simulink model "li_slotine"  (R2020b)
settings: Solver=VariableStepAuto  StartTime=0.0  StopTime=80  RelTol=1e-3
InitFcn:
  | UR5_LI_SLOTINE
values from neighbouring files (symbols this model uses):
  init_cond_regress = zeros(60, 1)    [UR5_LI_SLOTINE.m]    (also in parametersUR5_ADAPTIVE_BACKSTEPPING.m)
  init_config = [0,-55.5,-131,-2.5,20,105]'*pi/180    [UR5_LI_SLOTINE.m]    (also in parametersUR5_ADAPTIVE_BACKSTEPPING.m = [0,-37,-110,-2.5,-1,55]'*pi/180; parametersUR5_BACKSTEPPING.m = [0,-37,-110,-2.5,-1,55]'*pi/180)
  m1 = ur5.links(1,1).m    [UR5_LI_SLOTINE.m]    (also in parametersUR5_ADAPTIVE_BACKSTEPPING.m; parametersUR5_BACKSTEPPING.m)
  m2 = ur5.links(1,2).m    [UR5_LI_SLOTINE.m]    (also in parametersUR5_ADAPTIVE_BACKSTEPPING.m; parametersUR5_BACKSTEPPING.m)
  m3 = ur5.links(1,3).m    [UR5_LI_SLOTINE.m]    (also in parametersUR5_ADAPTIVE_BACKSTEPPING.m; parametersUR5_BACKSTEPPING.m)
  m4 = ur5.links(1,4).m    [UR5_LI_SLOTINE.m]    (also in parametersUR5_ADAPTIVE_BACKSTEPPING.m; parametersUR5_BACKSTEPPING.m)
  m5 = ur5.links(1,5).m    [UR5_LI_SLOTINE.m]    (also in parametersUR5_ADAPTIVE_BACKSTEPPING.m; parametersUR5_BACKSTEPPING.m)
  m6 = ur5.links(1,6).m    [UR5_LI_SLOTINE.m]    (also in parametersUR5_ADAPTIVE_BACKSTEPPING.m; parametersUR5_BACKSTEPPING.m)
  Ts = 1/100    (= 0.01)    [UR5_LI_SLOTINE.m]    (also in parametersUR5_ADAPTIVE_BACKSTEPPING.m; parametersUR5_BACKSTEPPING.m)
libraries: simulink x3, robotcorelib x1, cstblocks x1
settings Model: Creator=stefa  LastModifiedBy=stefa

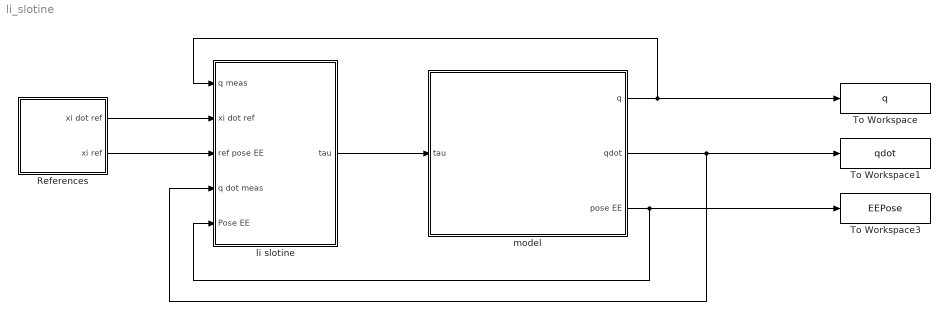
== system li_slotine ==
  References : Subsystem
  To Workspace : ToWorkspace  VariableName=q  SaveFormat=Timeseries  SampleTime=Ts
  To Workspace1 : ToWorkspace  VariableName=qdot  SaveFormat=Timeseries  SampleTime=Ts
  To Workspace3 : ToWorkspace  VariableName=EEPose  SaveFormat=Timeseries  SampleTime=Ts
  li slotine : Subsystem  StopFcn=show_results
  model : Subsystem
  wires:
  li slotine/1(tau) -> model/1(tau)
  model/1(q) -> li slotine/1(q meas), To Workspace/1
  model/2(qdot) -> li slotine/4(q dot meas), To Workspace1/1
  model/3(pose EE) -> li slotine/5(Pose EE), To Workspace3/1
  References/2(xi ref) -> li slotine/3(ref pose EE)
  References/1(xi dot ref) -> li slotine/2(xi dot ref)

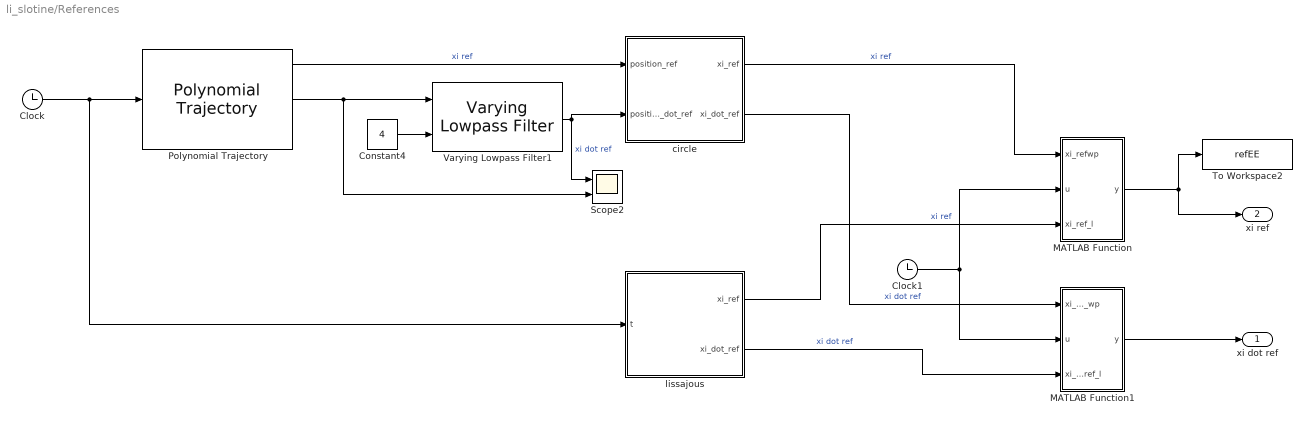
== system li_slotine/References ==
  Clock : Clock
  Clock1 : Clock
  Constant4 : Constant  Value=4
  MATLAB Function : MATLAB Function  TreatAsAtomicUnit=on
  MATLAB Function1 : MATLAB Function  TreatAsAtomicUnit=on
  Polynomial Trajectory : robotcorelib/Polynomial Trajectory  WaypointSource=Internal  Waypoints=waypoints  TimePoints=timepoints  TimeInterval=[ 1, 4 ]  Method=Cubic Polynomial  ParameterSource=Internal  VelocityBoundaryCondition=velocitybc  AccelerationBoundaryCondition=zeros( 2, 5 )  SimulateUsing=Interpreted execution
  Scope2 : Scope  NumInputPorts=2
  To Workspace2 : ToWorkspace  VariableName=refEE  SaveFormat=Timeseries  SampleTime=Ts
  Varying Lowpass Filter1 : cstblocks/Linear Parameter Varying/Varying Lowpass Filter  N=1
  circle : MATLAB Function  TreatAsAtomicUnit=on
  lissajous : MATLAB Function  TreatAsAtomicUnit=on
  xi dot ref : Outport
  xi ref : Outport  Port=2
  wires:
  lissajous/2(xi_dot_ref) -> MATLAB Function1/3(xi_dot_ref_l)  "xi dot ref"
  Polynomial Trajectory/2 -> Scope2/2, Varying Lowpass Filter1/1
  Constant4/1 -> Varying Lowpass Filter1/2
  circle/2(xi_dot_ref) -> MATLAB Function1/1(xi_dot_ref_wp)  "xi dot ref"
  Varying Lowpass Filter1/1 -> Scope2/1, circle/2(position_dot_ref)  "xi dot ref"
  circle/1(xi_ref) -> MATLAB Function/1(xi_refwp)  "xi ref"
  Clock/1 -> lissajous/1(t), Polynomial Trajectory/1
  Polynomial Trajectory/1 -> circle/1(position_ref)  "xi ref"
  lissajous/1(xi_ref) -> MATLAB Function/3(xi_ref_l)  "xi ref"
  MATLAB Function/1(y) -> xi ref/1, To Workspace2/1
  MATLAB Function1/1(y) -> xi dot ref/1
  Clock1/1 -> MATLAB Function1/2(u), MATLAB Function/2(u)

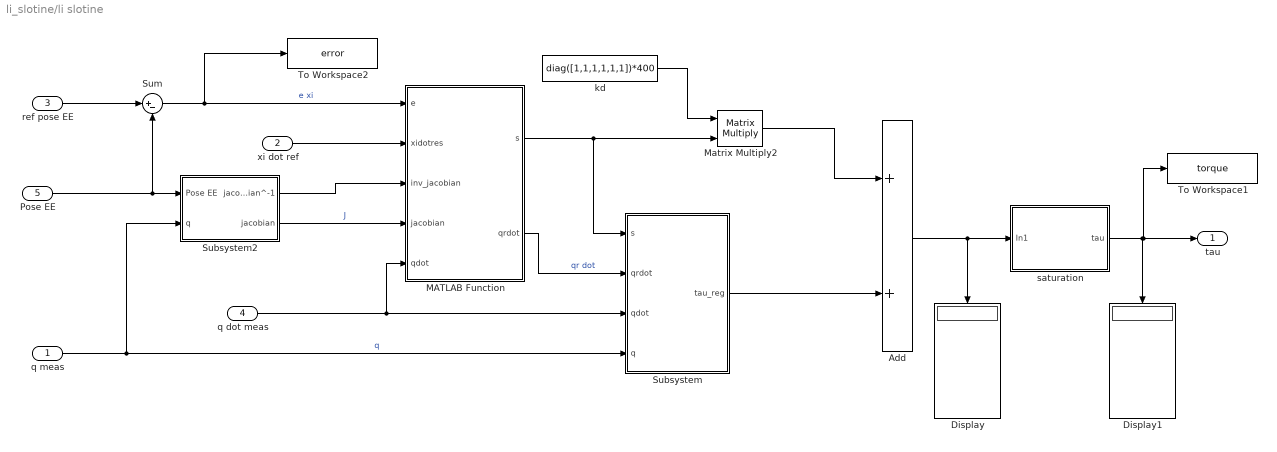
== system li_slotine/li slotine ==
  q meas : Inport
  xi dot ref : Inport  Port=2
  ref pose EE : Inport  Port=3
  q dot meas : Inport  Port=4
  Pose EE : Inport  Port=5
  Add : Sum
  Display : Display
  Display1 : Display
  MATLAB Function : MATLAB Function  TreatAsAtomicUnit=on
  Matrix Multiply2 : Product  Multiplication=Matrix(*)
  Subsystem : Subsystem
  Subsystem2 : Subsystem
  Sum : Sum  Inputs=|+-
  To Workspace1 : ToWorkspace  VariableName=torque  SaveFormat=Timeseries  SampleTime=Ts
  To Workspace2 : ToWorkspace  VariableName=error  SaveFormat=Timeseries  SampleTime=Ts
  kd : Constant  Value=diag([1,1,1,1,1,1])*400
  saturation : Subsystem
  tau : Outport
  wires:
  Add/1 -> saturation/1(In1), Display/1
  q meas/1 -> Subsystem/4(q), Subsystem2/2(q)  "q"
  MATLAB Function/2(qrdot) -> Subsystem/2(qrdot)  "qr dot"
  q dot meas/1 -> Subsystem/3(qdot), MATLAB Function/5(qdot)
  ref pose EE/1 -> Sum/1
  Pose EE/1 -> Sum/2, Subsystem2/1(Pose EE)
  Sum/1 -> To Workspace2/1, MATLAB Function/1(e)  "e xi"
  Subsystem2/1(jacobian^-1) -> MATLAB Function/3(inv_jacobian)
  Subsystem2/2(jacobian) -> MATLAB Function/4(jacobian)  "J"
  MATLAB Function/1(s) -> Subsystem/1(s), Matrix Multiply2/2
  Matrix Multiply2/1 -> Add/1
  kd/1 -> Matrix Multiply2/1
  xi dot ref/1 -> MATLAB Function/2(xidotres)
  Subsystem/1(tau_reg) -> Add/2
  saturation/1(tau) -> tau/1, To Workspace1/1, Display1/1

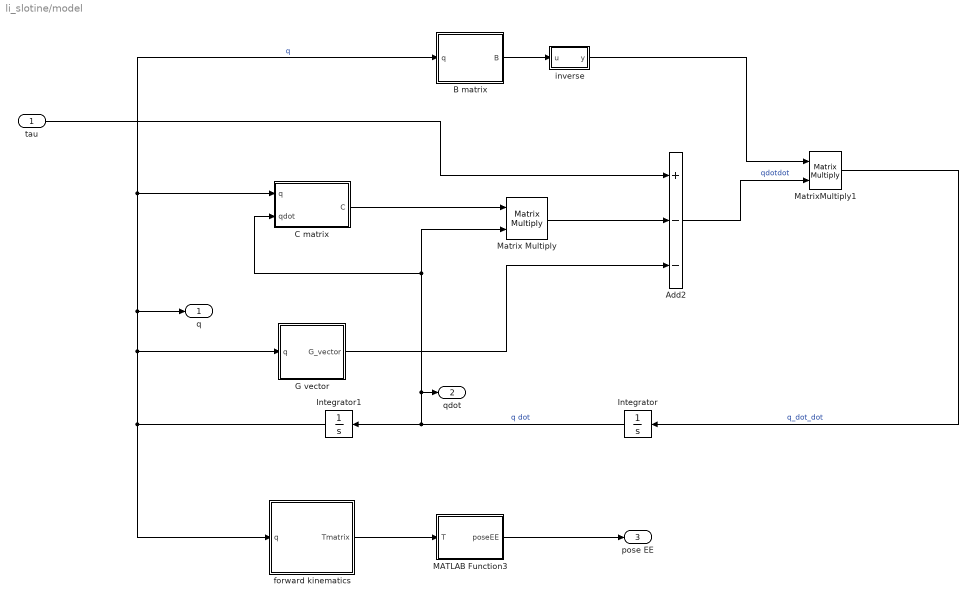
== system li_slotine/model ==
  tau : Inport
  Add2 : Sum  Inputs=+--
  B matrix : MATLAB Function  TreatAsAtomicUnit=on
  C matrix : MATLAB Function  TreatAsAtomicUnit=on
  G vector : MATLAB Function  TreatAsAtomicUnit=on
  Integrator : Integrator  InitialCondition=[0,0,0,0,0,0]'
  Integrator1 : Integrator  InitialCondition=init_config
  MATLAB Function3 : MATLAB Function  TreatAsAtomicUnit=on
  Matrix Multiply : Product  Multiplication=Matrix(*)
  MatrixMultiply1 : Product  Multiplication=Matrix(*)
  forward kinematics : MATLAB Function  TreatAsAtomicUnit=on
  inverse : MATLAB Function  TreatAsAtomicUnit=on
  q : Outport
  qdot : Outport  Port=2
  pose EE : Outport  Port=3
  wires:
  MatrixMultiply1/1 -> Integrator/1  "q_dot_dot"
  B matrix/1(B) -> inverse/1(u)
  inverse/1(y) -> MatrixMultiply1/1
  tau/1 -> Add2/1
  Matrix Multiply/1 -> Add2/2
  C matrix/1(C) -> Matrix Multiply/1
  Integrator/1 -> C matrix/2(qdot), Matrix Multiply/2, qdot/1, Integrator1/1  "q dot"
  Integrator1/1 -> G vector/1(q), q/1, B matrix/1(q), C matrix/1(q), forward kinematics/1(q)  "q"
  G vector/1(G_vector) -> Add2/3
  Add2/1 -> MatrixMultiply1/2  "qdotdot"
  forward kinematics/1(Tmatrix) -> MATLAB Function3/1(T)
  MATLAB Function3/1(poseEE) -> pose EE/1

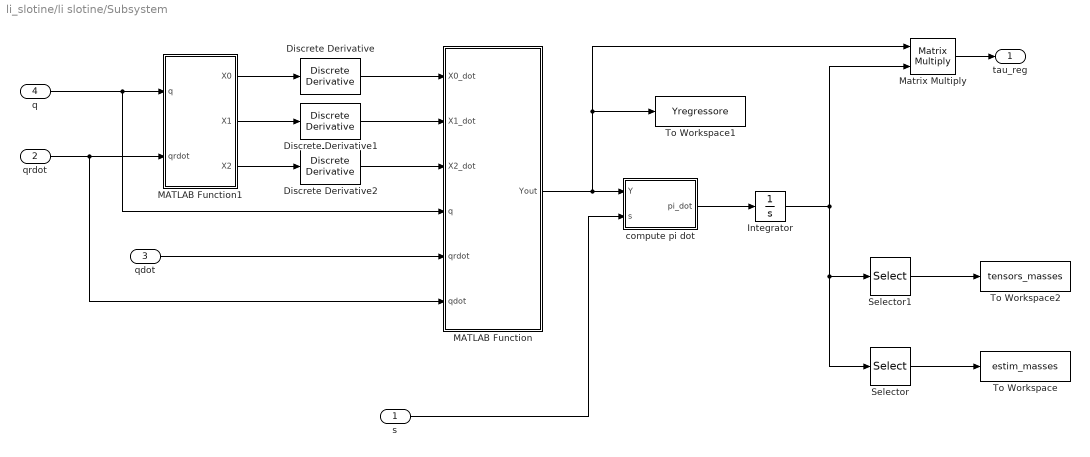
== system li_slotine/li slotine/Subsystem ==
  s : Inport
  qrdot : Inport  Port=2
  qdot : Inport  Port=3
  q : Inport  Port=4
  Discrete Derivative : simulink/Discrete/Discrete Derivative  gainval=1.0  ICPrevScaledInput=0.0  OutMin=[]  OutMax=[]  OutDataType=fixdt(1, 16)  OutScaling=2^-10  DoSatur=off
  Discrete Derivative1 : simulink/Discrete/Discrete Derivative  gainval=1.0  ICPrevScaledInput=0.0  OutMin=[]  OutMax=[]  OutDataType=fixdt(1, 16)  OutScaling=2^-10  DoSatur=off
  Discrete Derivative2 : simulink/Discrete/Discrete Derivative  gainval=1.0  ICPrevScaledInput=0.0  OutMin=[]  OutMax=[]  OutDataType=fixdt(1, 16)  OutScaling=2^-10  DoSatur=off
  Integrator : Integrator  InitialCondition=init_cond_regress
  MATLAB Function : MATLAB Function  TreatAsAtomicUnit=on
  MATLAB Function1 : MATLAB Function  TreatAsAtomicUnit=on
  Matrix Multiply : Product  Multiplication=Matrix(*)
  Selector : Selector  InputPortWidth=60  IndexOptions=Index vector (dialog)  Indices=[1:6]  OutputSizes=1
  Selector1 : Selector  InputPortWidth=60  IndexOptions=Index vector (dialog)  Indices=[25:60]  OutputSizes=1
  To Workspace : ToWorkspace  VariableName=estim_masses  SaveFormat=Timeseries  SampleTime=Ts
  To Workspace1 : ToWorkspace  VariableName=Yregressore  SaveFormat=Timeseries  SampleTime=Ts
  To Workspace2 : ToWorkspace  VariableName=tensors_masses  SaveFormat=Timeseries  SampleTime=Ts
  compute pi dot : MATLAB Function  TreatAsAtomicUnit=on
  tau_reg : Outport
  wires:
  q/1 -> MATLAB Function/4(q), MATLAB Function1/1(q)
  qrdot/1 -> MATLAB Function/6(qdot), MATLAB Function1/2(qrdot)
  MATLAB Function1/1(X0) -> Discrete Derivative/1
  MATLAB Function1/2(X1) -> Discrete Derivative1/1
  MATLAB Function1/3(X2) -> Discrete Derivative2/1
  Discrete Derivative/1 -> MATLAB Function/1(X0_dot)
  Discrete Derivative1/1 -> MATLAB Function/2(X1_dot)
  Discrete Derivative2/1 -> MATLAB Function/3(X2_dot)
  qdot/1 -> MATLAB Function/5(qrdot)
  MATLAB Function/1(Yout) -> Matrix Multiply/1, To Workspace1/1, compute pi dot/1(Y)
  compute pi dot/1(pi_dot) -> Integrator/1
  s/1 -> compute pi dot/2(s)
  Integrator/1 -> Selector/1, Selector1/1, Matrix Multiply/2
  Matrix Multiply/1 -> tau_reg/1
  Selector/1 -> To Workspace/1
  Selector1/1 -> To Workspace2/1

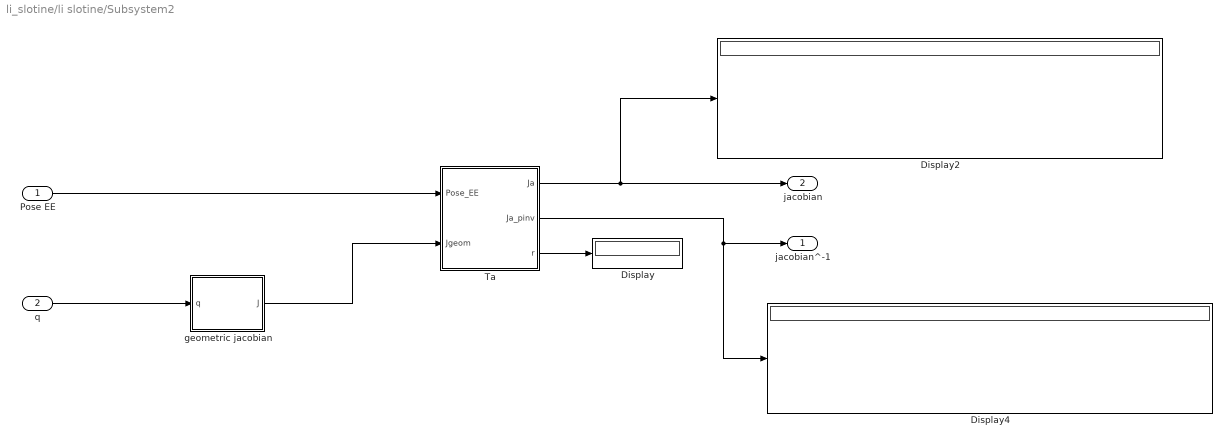
== system li_slotine/li slotine/Subsystem2 ==
  Pose EE : Inport
  q : Inport  Port=2
  Display : Display
  Display2 : Display
  Display4 : Display
  Ta : MATLAB Function  TreatAsAtomicUnit=on
  geometric jacobian : MATLAB Function  TreatAsAtomicUnit=on
  jacobian^-1 : Outport
  jacobian : Outport  Port=2
  wires:
  Pose EE/1 -> Ta/1(Pose_EE)
  q/1 -> geometric jacobian/1(q)
  Ta/2(Ja_pinv) -> jacobian^-1/1, Display4/1
  Ta/1(Ja) -> jacobian/1, Display2/1
  Ta/3(r) -> Display/1
  geometric jacobian/1(J) -> Ta/2(Jgeom)

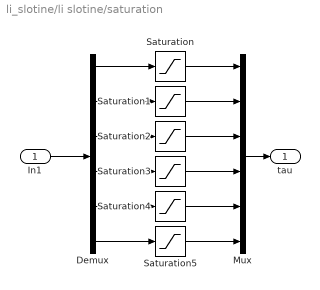
== system li_slotine/li slotine/saturation ==
  In1 : Inport
  Demux : Demux  Outputs=6
  Mux : Mux  Inputs=6
  Saturation : Saturate  UpperLimit=150  LowerLimit=-150
  Saturation1 : Saturate  UpperLimit=150  LowerLimit=-150
  Saturation2 : Saturate  UpperLimit=150  LowerLimit=-150
  Saturation3 : Saturate  UpperLimit=28  LowerLimit=-28
  Saturation4 : Saturate  UpperLimit=28  LowerLimit=-28
  Saturation5 : Saturate  UpperLimit=28  LowerLimit=-28
  tau : Outport
  wires:
  In1/1 -> Demux/1
  Mux/1 -> tau/1
  Demux/1 -> Saturation/1
  Demux/2 -> Saturation1/1
  Demux/3 -> Saturation2/1
  Demux/4 -> Saturation3/1
  Demux/5 -> Saturation4/1
  Demux/6 -> Saturation5/1
  Saturation/1 -> Mux/1
  Saturation1/1 -> Mux/2
  Saturation2/1 -> Mux/3
  Saturation3/1 -> Mux/4
  Saturation4/1 -> Mux/5
  Saturation5/1 -> Mux/6

== matlab function li_slotine/model/forward kinematics ==
  data: q input; Tmatrix output
function Tmatrix = fkine(q)
%#codegen

%    This function was generated by the Symbolic Math Toolbox version 8.6.
%    20-Jan-2022 14:28:01

q1 = q(1);
q2 = q(2);
q3 = q(3);
q4 = q(4);
q5 = q(5);
q6 = q(6);
t2 = cos(q1);
t3 = cos(q2);
t4 = cos(q3);
t5 = cos(q4);
t6 = cos(q5);
t7 = cos(q6);
t8 = sin(q1);
t9 = sin(q2);
t10 = sin(q3);
t11 = sin(q4);
t12 = sin(q5);
t13 = sin(q6);
t14 = q2+q3;
t23 = cos(1.570796327);
t24 = sin(1.570796327);
t25 = sin(3.141592654);
t15 = q4+t14;
t16 = t2.*t3;
t18 = t2.*t9;
t19 = t3.*t8;
t21 = t8.*t9;
t26 = t23.^2;
t27 = t24.^2;
t58 = t2.*t23.*t24;
t59 = t8.*t23.*t24;
t17 = cos(t15);
t20 = sin(t15);
t28 = t16.*t23;
t29 = t18.*t23;
t30 = t19.*t23;
t31 = t21.*t23;
t32 = t2.*t27;
t33 = t8.*t27;
t38 = t3.*t4.*t5.*t27;
t39 = t3.*t10.*t11.*t27;
t40 = t4.*t9.*t11.*t27;
t41 = t5.*t9.*t10.*t27;
t60 = -t58;
t22 = t17+1.0;
t34 = -t28;
t35 = -t31;
t36 = -t33;
t37 = t6.*t20.*t24;
t42 = -t38;
t43 = t18+t30;
t44 = t19+t29;
t61 = t12.*t20.*t23.*t24;
t45 = t16+t35;
t46 = t21+t34;
t47 = (t12.*t22.*t25)./2.0;
t48 = t4.*t43;
t49 = t4.*t44;
t50 = t10.*t43;
t51 = t10.*t44;
t62 = (t6.*t22.*t23.*t25)./2.0;
t85 = t26+t39+t40+t41+t42;
t52 = t4.*t45;
t53 = t4.*t46;
t54 = t10.*t45;
t55 = t10.*t46;
t56 = -t50;
t63 = -t62;
t64 = t37+t47;
t89 = t24.*t85;
t57 = -t55;
t65 = t48+t54;
t66 = t51+t53;
t68 = t52+t56;
t72 = -t5.*(t50-t52);
t80 = -t11.*t23.*(t50-t52);
t82 = -t11.*t24.*(t50-t52);
t103 = t61+t63+t89;
t67 = t49+t57;
t69 = t11.*t65;
t70 = t11.*t66;
t75 = t5.*t23.*t65;
t76 = t5.*t23.*t66;
t77 = t5.*t24.*t65;
t78 = t5.*t24.*t66;
t71 = t5.*t67;
t73 = -t69;
t74 = -t70;
t79 = t11.*t23.*t67;
t81 = t11.*t24.*t67;
t87 = -t6.*(t69+t5.*(t50-t52));
t91 = -t12.*t23.*(t69+t5.*(t50-t52));
t93 = t36+t75+t80;
t97 = t59+t77+t82;
t83 = t71+t74;
t84 = t72+t73;
t86 = -t6.*(t70-t71);
t88 = t6.*(t70-t71);
t90 = -t12.*t23.*(t70-t71);
t92 = t32+t76+t79;
t95 = t12.*t93;
t98 = t60+t78+t81;
t100 = t6.*t23.*t93;
t101 = t24.*t97;
t94 = t12.*t92;
t96 = -t95;
t99 = t6.*t23.*t92;
t102 = t24.*t98;
t107 = t91+t100+t101;
t104 = t88+t94;
t105 = t87+t96;
t106 = t90+t99+t102;
Tmatrix = reshape([-t13.*t107-t7.*(t95+t6.*(t69+t5.*(t50-t52))),-t7.*t104-t13.*t106,t7.*t64-t13.*t103,0.0,-t7.*t107+t13.*(t95+t6.*(t69+t5.*(t50-t52))),-t7.*t106+t13.*t104,-t13.*t64-t7.*t103,0.0,t23.*t97+t12.*t24.*(t69+t5.*(t50-t52))-t6.*t24.*t93,t23.*t98-t6.*t24.*t92+t12.*t24.*(t70-t71),t23.*t85-t12.*t20.*t27+(t6.*t22.*t24.*t25)./2.0,0.0,t16.*(-1.7e+1./4.0e+1)+t31.*(1.7e+1./4.0e+1)+t50.*3.9225e-1-t52.*3.9225e-1+t59.*9.465e-2+t77.*9.465e-2+t8.*t24.*1.0915e-1+t23.*t97.*8.23e-2+t12.*t24.*(t69+t5.*(t50-t52)).*8.23e-2-t6.*t24.*t93.*8.23e-2-t11.*t24.*(t50-t52).*9.465e-2,t19.*(-1.7e+1./4.0e+1)-t29.*(1.7e+1./4.0e+1)-t49.*3.9225e-1+t55.*3.9225e-1-t58.*9.465e-2+t78.*9.465e-2+t81.*9.465e-2-t2.*t24.*1.0915e-1+t23.*t98.*8.23e-2-t6.*t24.*t92.*8.23e-2+t12.*t24.*(t70-t71).*8.23e-2,t23.*1.0915e-1+t26.*9.465e-2-t9.*t24.*(1.7e+1./4.0e+1)-t23.*t38.*8.23e-2+t23.*t39.*8.23e-2+t23.*t40.*8.23e-2+t23.*t41.*8.23e-2+t23.^3.*8.23e-2-t5.*t27.*cos(t14).*9.465e-2+t11.*t27.*sin(t14).*9.465e-2-t3.*t10.*t24.*3.9225e-1-t4.*t9.*t24.*3.9225e-1+t6.*t24.*t25.*4.115e-2-t12.*t20.*t27.*8.23e-2+t6.*t17.*t24.*t25.*4.115e-2+8.9459e-2,1.0],[4,4]);

== matlab function li_slotine/li slotine/Subsystem2/Ta ==
  data: Pose_EE input; Ja output; Ja_pinv output; Jgeom input; r output
function [Ja, Ja_pinv, r ]= fcn(Pose_EE, Jgeom)
Ja=zeros(6,6);
Ja_pinv=zeros(6,6);

phi = Pose_EE(4);
theta = Pose_EE(5);

%% con ZYZ
Ta = [0     -sin(phi)       cos(phi)*sin(theta) ;
      0      cos(phi)       sin(phi)*sin(theta) ;
      1          0                    cos(theta)];


Ja = inv([eye(3), zeros(3); zeros(3), Ta]) * Jgeom;

%Ja_pinv = inv(Ja);
Ja_pinv = pinv(Ja, 0.0005);
%Ja_pinv = damped_pseudo_inverse(Ja,0.1,0.1);
r = rank(Ja);

end

== matlab function li_slotine/li slotine/Subsystem/MATLAB Function ==
  data: X0_dot input; Yout output; X1_dot input; X2_dot input; q input; qrdot input; qdot input
function Yout = fcn(X0_dot, X1_dot, X2_dot, q, qrdot, qdot)
Y_1 = zeros(6,10);
Y_2 = zeros(6,10);
Y_3 = zeros(6,10);
Y_4 = zeros(6,10);
Y_5 = zeros(6,10);
Y_6 = zeros(6,10);
Yout = zeros(6, 60);

q1 = q(1);
q2 = q(2);
q3 = q(3);
q4 = q(4);
q5 = q(5);
q6 = q(6);

q1rdot = qrdot(1);
q2rdot = qrdot(2);
q3rdot = qrdot(3);
q4rdot = qrdot(4);
q5rdot = qrdot(5);
q6rdot = qrdot(6);

q1dot = qdot(1);
q2dot = qdot(2);
q3dot = qdot(3);
q4dot = qdot(4);
q5dot = qdot(5);
q6dot = qdot(6);

Y0_1 = X0_dot(:,1) - W0_1_mat + Z0_1_mat;
Y0_2 = X0_dot(:,2) - W0_2_mat(q1,q2,q1dot,q2dot,q1rdot,q2rdot) + Z0_2_mat(q1,q2);
Y0_3 = X0_dot(:,3) - W0_3_mat(q1,q2,q3,q1dot,q2dot,q3dot,q1rdot,q2rdot,q3rdot) + Z0_3_mat(q1,q2,q3);
Y0_4 = X0_dot(:,4) - W0_4_mat(q1,q2,q3,q1dot,q2dot,q3dot,q1rdot,q2rdot,q3rdot) + Z0_4_mat(q1,q2,q3);
Y0_5 = X0_dot(:,5) - W0_5_mat(q1,q2,q3,q4,q1dot,q2dot,q3dot,q4dot,q5dot,q1rdot,q2rdot,q3rdot,q4rdot,q5rdot) + Z0_5_mat(q1,q2,q3,q4);
Y0_6 = X0_dot(:,6) - W0_6_mat(q1,q2,q3,q4,q5,q1dot,q2dot,q3dot,q4dot,q5dot,q6dot,q1rdot,q2rdot,q3rdot,q4rdot,q5rdot,q6rdot) + Z0_6_mat(q1,q2,q3,q4,q5);

Y1_1 = X1_dot(:,1:3) - W1_1_mat + Z1_1_mat;
Y1_2 = X1_dot(:,4:6) - W1_2_mat(q1,q2,q1dot,q2dot,q1rdot,q2rdot) + Z1_2_mat(q2);
Y1_3 = X1_dot(:,7:9) - W1_3_mat(q1,q2,q3,q1dot,q2dot,q3dot,q1rdot,q2rdot,q3rdot) + Z1_3_mat(q2,q3);
Y1_4 = X1_dot(:,10:12) - W1_4_mat(q1,q2,q3,q4,q1dot,q2dot,q3dot,q4dot,q1rdot,q2rdot,q3rdot,q4rdot) + Z1_4_mat(q2,q3,q4);
Y1_5 = X1_dot(:,13:15) - W1_5_mat(q1,q2,q3,q4,q5,q1dot,q2dot,q3dot,q4dot,q5dot,q1rdot,q2rdot,q3rdot,q4rdot,q5rdot) + Z1_5_mat(q2,q3,q4,q5);
Y1_6 = X1_dot(:,16:18) - W1_6_mat(q1,q2,q3,q4,q5,q6,q1dot,q2dot,q3dot,q4dot,q5dot,q6dot,q1rdot,q2rdot,q3rdot,q4rdot,q5rdot,q6rdot) + Z1_6_mat(q2,q3,q4,q5,q6);

Y2_1 = X2_dot(:,1:6) - W2_1_mat;
Y2_2 = X2_dot(:,7:12) - W2_2_mat(q2,q1dot,q2dot);
Y2_3 = X2_dot(:,13:18) - W2_3_mat(q2,q3,q1dot,q2dot,q3dot);
Y2_4 = X2_dot(:,19:24) - W2_4_mat(q2,q3,q4,q1dot,q2dot,q3dot,q4dot);
Y2_5 = X2_dot(:,25:30) - W2_5_mat(q2,q3,q4,q5,q1dot,q2dot,q3dot,q4dot,q5dot);
Y2_6 = X2_dot(:,31:36) - W2_6_mat(q2,q3,q4,q5,q6,q1dot,q2dot,q3dot,q4dot,q5dot,q6dot);

Y_1 = [Y0_1, Y1_1, Y2_1]; % 6x1, 6x3, 6x6
Y_2 = [Y0_2, Y1_2, Y2_2];
Y_3 = [Y0_3, Y1_3, Y2_3];
Y_4 = [Y0_4, Y1_4, Y2_4];
Y_5 = [Y0_5, Y1_5, Y2_5];
Y_6 = [Y0_6, Y1_6, Y2_6];


Yout = [Y_1, Y_2, Y_3, Y_4, Y_5, Y_6];
end

== matlab function li_slotine/li slotine/Subsystem/compute pi dot ==
  data: Y input; pi_dot output; s input
function pi_dot = fcn(Y, s)

R = 0.1*eye(60);
%R = 0.1*eye(60);

pi_dot = inv(R)*Y'*s;

== matlab function li_slotine/References/lissajous ==
  data: t input; xi_ref output; xi_dot_ref output
function [xi_ref,xi_dot_ref] = fcn(t)
    xi_ref = zeros(6,1);
    xi_dot_ref = zeros(6,1);

    initial_position = [-0.0597   -0.1914    0.6397];
    initial_orientation = [1.5558   -1.5797    3.0630]';
    A =0.15;
    metodo_di_slow = 0.1;
    p = 3;
    q = 2;
    
    t = t - 10;
    
    x = A*sin(p*t*metodo_di_slow +pi/2) + initial_position(1)-A;
    y = initial_position(2);
    z = A*sin(q*t*metodo_di_slow ) + initial_position(3);

    xdot = -p*A*sin(p*t*metodo_di_slow )*metodo_di_slow ;
    ydot = 0;
    zdot = q*A * cos(q*t*metodo_di_slow )*metodo_di_slow ;

    

    position_ref = [x,y,z]';
    position_dot_ref =[xdot, ydot, zdot]';
    
    xi_ref = [position_ref ; initial_orientation];
    xi_dot_ref = [position_dot_ref ; 0;    0  ; 0];

== matlab function li_slotine/References/circle ==
  data: position_ref input; xi_ref output; xi_dot_ref output; position_dot_ref input
function [xi_ref,xi_dot_ref] = fcn(position_ref, position_dot_ref)
    xi_ref = zeros(6,1);
    xi_dot_ref = zeros(6,1);
    
    
    %initial_orientation = [1.5558   -1.5797    3.0630]'; se partiamo
    %dall'inizio della traiettoria di l
    initial_orientation = [1.9159   -1.6243   -3.0275]';
    
    
    xi_ref = [position_ref ; initial_orientation];
    xi_dot_ref = [position_dot_ref ; 0;    0  ; 0];

== matlab function li_slotine/model/inverse ==
  data: u input; y output
function y = fcn(u)

y = inv(u);

== matlab function li_slotine/li slotine/Subsystem2/geometric jacobian ==
  data: q input; J output
function J = jacob0(q)

J = Jacobian0(q(1),q(2),q(3),q(4),q(5),q(6));

== matlab function li_slotine/model/MATLAB Function3 ==
  data: T input; poseEE output
function poseEE = fcn(T)
    poseEE = zeros(6,1);
    coder.extrinsic('tform2eul');
    
    O = [0; 0; 0];        % world origin frame

    position = T * [O; 1];
    orientation = tform2eul(T, 'ZYZ');

    poseEE = [position(1:3); orientation'];
end

== matlab function li_slotine/References/MATLAB Function ==
  data: xi_refwp input; u input; xi_ref_l input; y output
function y = fcn(xi_refwp, u, xi_ref_l)

if u < 10
    y = xi_refwp;
else
    y = xi_ref_l;
end

== matlab function li_slotine/model/B matrix ==
  data: q input; B output; m1 parameter; m2 parameter; m3 parameter; m4 parameter; m5 parameter; m6 parameter
function B = fcn(q, m1, m2, m3, m4, m5, m6)

B = Mmatrix(m1,m2,m3,m4,m5,m6,q(2),q(3),q(4),q(5));

== matlab function li_slotine/References/MATLAB Function1 ==
  data: xi_dot_ref_wp input; u input; y output; xi_dot_ref_l input
function y = fcn(xi_dot_ref_wp, u, xi_dot_ref_l)

if u < 10
    y = xi_dot_ref_wp;
else
    y = xi_dot_ref_l;
end

== matlab function li_slotine/li slotine/MATLAB Function ==
  data: s output; e input; xidotres input; inv_jacobian input; jacobian input; qdot input; qrdot output
function [s, qrdot] = fcn(e, xidotres, inv_jacobian, jacobian, qdot)

lambda = 2*diag([1,150,150,0.8,0.6,1]);   % se non siamo sul punto iniziale della traiettoria

%    lambda =110*diag([1,1,1,0.8,0.1,0.01]);  % se siamo sul punto iniziale della traiettoria

edot = xidotres - jacobian*(qdot);

s = inv_jacobian * (edot + lambda * e);

qrdot = s + qdot;

%eJt = jacobian'*e;

== matlab function li_slotine/model/C matrix ==
  data: q input; C output; qdot input; m2 parameter; m3 parameter; m4 parameter; m5 parameter; m6 parameter
function C = C_matrix(q, qdot, m2, m3, m4, m5, m6)

C = Cmatrix(m2,m3,m4,m5,m6,q(2),q(3),q(4),q(5),qdot(1),qdot(2),qdot(3),qdot(4),qdot(5),qdot(6));

== matlab function li_slotine/model/G vector ==
  data: q input; G_vector output; m2 parameter; m3 parameter; m4 parameter; m5 parameter; m6 parameter
function G_vector = gravload(q, m2, m3, m4, m5, m6)

G_vector = Gvector(m2,m3,m4,m5,m6,q(2),q(3),q(4),q(5))';

== matlab function li_slotine/li slotine/Subsystem/MATLAB Function1 ==
  data: X0 output; X1 output; X2 output; q input; qrdot input
function [X0, X1, X2] = getX(q, qrdot)

q1 = q(1);
q2 = q(2);
q3 = q(3);
q4 = q(4);
q5 = q(5);
q6 = q(6);

q1rdot = qrdot(1);
q2rdot = qrdot(2);
q3rdot = qrdot(3);
q4rdot = qrdot(4);
q5rdot = qrdot(5);
q6rdot = qrdot(6);


X0 = zeros(6,6);
X1 = zeros(6,18);
X2 = zeros(6,36);

X0_1_s = X0_1_mat;
X0_2_s = X0_2_mat(q1,q2,q1rdot,q2rdot);
X0_3_s = X0_3_mat(q1,q2,q3,q1rdot,q2rdot,q3rdot);
X0_4_s = X0_4_mat(q1,q2,q3,q1rdot,q2rdot,q3rdot);
X0_5_s = X0_5_mat(q1,q2,q3,q4,q1rdot,q2rdot,q3rdot,q4rdot,q5rdot);
X0_6_s = X0_6_mat(q1,q2,q3,q4,q5,q1rdot,q2rdot,q3rdot,q4rdot,q5rdot,q6rdot);

X0 = [X0_1_s, X0_2_s, X0_3_s, X0_4_s, X0_5_s, X0_6_s];

X1_1_s = X1_1_mat;
X1_2_s = X1_2_mat(q1,q2,q1rdot,q2rdot);
X1_3_s = X1_3_mat(q1,q2,q3,q1rdot,q2rdot,q3rdot);
X1_4_s = X1_4_mat(q1,q2,q3,q4,q1rdot,q2rdot,q3rdot,q4rdot);
X1_5_s = X1_5_mat(q1,q2,q3,q4,q5,q1rdot,q2rdot,q3rdot,q4rdot,q5rdot);
X1_6_s = X1_6_mat(q1,q2,q3,q4,q5,q6,q1rdot,q2rdot,q3rdot,q4rdot,q5rdot,q6rdot);

X1 = [X1_1_s, X1_2_s, X1_3_s, X1_4_s, X1_5_s, X1_6_s];

X2_1_s = X2_1_mat(q1rdot);
X2_2_s = X2_2_mat(q1,q2,q1rdot,q2rdot);
X2_3_s = X2_3_mat(q1,q2,q3,q1rdot,q2rdot,q3rdot);
X2_4_s = X2_4_mat(q1,q2,q3,q4,q1rdot,q2rdot,q3rdot,q4rdot);
X2_5_s = X2_5_mat(q1,q2,q3,q4,q5,q1rdot,q2rdot,q3rdot,q4rdot,q5rdot);
X2_6_s = X2_6_mat(q1,q2,q3,q4,q5,q6,q1rdot,q2rdot,q3rdot,q4rdot,q5rdot,q6rdot);

X2 = [X2_1_s, X2_2_s, X2_3_s, X2_4_s, X2_5_s, X2_6_s];
